simulink model "LAB1__2_2"  (R2020a)
settings: Solver=VariableStepAuto  StartTime=0.0  StopTime=10.0  RelTol=1e-3
settings Model: Creator=Пользователь  LastModifiedBy=Пользователь

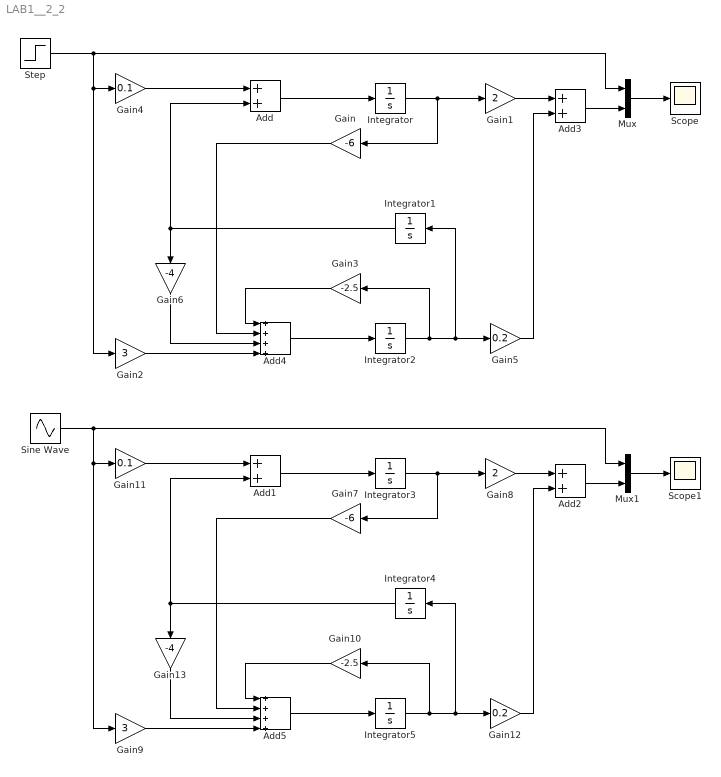
== system LAB1__2_2 ==
  Add{,1..3} (4 alike) : Sum
  Add4 : Sum  Inputs=++++
  Add5 : Sum  Inputs=++++
  Gain : Gain  Gain=-6
  Gain1 : Gain  Gain=2
  Gain10 : Gain  Gain=-2.5
  Gain11 : Gain  Gain=0.1
  Gain12 : Gain  Gain=0.2
  Gain13 : Gain  Gain=-4
  Gain2 : Gain  Gain=3
  Gain3 : Gain  Gain=-2.5
  Gain4 : Gain  Gain=0.1
  Gain5 : Gain  Gain=0.2
  Gain6 : Gain  Gain=-4
  Gain7 : Gain  Gain=-6
  Gain8 : Gain  Gain=2
  Gain9 : Gain  Gain=3
  Integrator{,1..5} (6 alike) : Integrator
  Mux : Mux  Inputs=2
  Mux1 : Mux  Inputs=2
  Scope : Scope
  Scope1 : Scope
  Sine Wave : Sin  Amplitude=2  SampleTime=0
  Step : Step  Time=0.5  SampleTime=0
  wires:
  Step/1 -> Gain2/1, Gain4/1, Mux/1
  Gain4/1 -> Add/1
  Add/1 -> Integrator/1
  Integrator/1 -> Gain/1, Gain1/1
  Gain1/1 -> Add3/1
  Add4/1 -> Integrator2/1
  Integrator2/1 -> Integrator1/1, Gain5/1, Gain3/1
  Integrator1/1 -> Add/2, Gain6/1
  Gain5/1 -> Add3/2
  Mux/1 -> Scope/1
  Add3/1 -> Mux/2
  Gain2/1 -> Add4/4
  Gain6/1 -> Add4/3
  Gain/1 -> Add4/2
  Gain3/1 -> Add4/1
  Gain7/1 -> Add5/2
  Add2/1 -> Mux1/2
  Mux1/1 -> Scope1/1
  Gain13/1 -> Add5/3
  Gain12/1 -> Add2/2
  Add5/1 -> Integrator5/1
  Gain10/1 -> Add5/1
  Integrator4/1 -> Add1/2, Gain13/1
  Integrator5/1 -> Integrator4/1, Gain12/1, Gain10/1
  Integrator3/1 -> Gain7/1, Gain8/1
  Gain8/1 -> Add2/1
  Sine Wave/1 -> Mux1/1, Gain9/1, Gain11/1
  Gain11/1 -> Add1/1
  Add1/1 -> Integrator3/1
  Gain9/1 -> Add5/4
